simulink model "ANCwithError"  (R2023b)
settings: Solver=VariableStepAuto  StartTime=0.0  StopTime=10.0  RelTol=1e-3
libraries: matrix_library x54, dspadpt3 x30, raspberrypiAVlib x2, dspfdesign x2, audiosources x1
(part 2 of 2)

== system ANCwithError/Audio Processing/Subsystem2/Subsystem4 ==
  In1 : Inport
  In2 : Inport  Port=2
  Constant : Constant  Value=0.5
  Delay1 : Delay  DelayLength=1
  Estim. sec. path : DiscreteFir  Commented=through  Coefficients="[0.466  0.533  -0.257  -0.274  -0.231  -0.175]"
  Gain : Gain  Gain=-1
  LMS Update : dspadpt3/LMS Update  Method=Normalized LMS  Length=200  NumFilters=1  StepSizeSource=Input port  StepSize=0.1  LeakageFactor=1.0  InitialConditions=0  AdaptiveFilterMode=Tapped delay-line FIR filter  EnableAdaptInput=off  EnableResetInput=off  SimulateUsing=Interpreted execution
  LMS filter copy : DiscreteFir  CoefSource=Input port
      settings: InputPortMap=u0,u1
  y : Outport
  wires:
  Gain/1 -> y/1
  Constant/1 -> LMS Update/3
  LMS filter copy/1 -> Gain/1
  [coefs] -> LMS filter copy/2
  Delay1/1 -> [coefs]
  LMS Update/1 -> Delay1/1
  In1/1 -> Estim. sec. path/1, LMS filter copy/1
  Estim. sec. path/1 -> LMS Update/1
  In2/1 -> LMS Update/2

== system ANCwithError/Audio Processing/Subsystem2/Subsystem5 ==
  In1 : Inport
  In2 : Inport  Port=2
  Constant : Constant  Value=0.5
  Delay1 : Delay  DelayLength=1
  Estim. sec. path : DiscreteFir  Commented=through  Coefficients="[0.466  0.533  -0.257  -0.274  -0.231  -0.175]"
  Gain : Gain  Gain=-1
  LMS Update : dspadpt3/LMS Update  Method=Normalized LMS  Length=200  NumFilters=1  StepSizeSource=Input port  StepSize=0.1  LeakageFactor=1.0  InitialConditions=0  AdaptiveFilterMode=Tapped delay-line FIR filter  EnableAdaptInput=off  EnableResetInput=off  SimulateUsing=Interpreted execution
  LMS filter copy : DiscreteFir  CoefSource=Input port
      settings: InputPortMap=u0,u1
  y : Outport
  wires:
  Gain/1 -> y/1
  Constant/1 -> LMS Update/3
  LMS filter copy/1 -> Gain/1
  [coefs] -> LMS filter copy/2
  Delay1/1 -> [coefs]
  LMS Update/1 -> Delay1/1
  In1/1 -> Estim. sec. path/1, LMS filter copy/1
  Estim. sec. path/1 -> LMS Update/1
  In2/1 -> LMS Update/2

== system ANCwithError/Audio Processing/Subsystem2/Subsystem6 ==
  In1 : Inport
  In2 : Inport  Port=2
  Constant : Constant  Value=0.5
  Delay1 : Delay  DelayLength=1
  Estim. sec. path : DiscreteFir  Commented=through  Coefficients="[0.466  0.533  -0.257  -0.274  -0.231  -0.175]"
  Gain : Gain  Gain=-1
  LMS Update : dspadpt3/LMS Update  Method=Normalized LMS  Length=200  NumFilters=1  StepSizeSource=Input port  StepSize=0.1  LeakageFactor=1.0  InitialConditions=0  AdaptiveFilterMode=Tapped delay-line FIR filter  EnableAdaptInput=off  EnableResetInput=off  SimulateUsing=Interpreted execution
  LMS filter copy : DiscreteFir  CoefSource=Input port
      settings: InputPortMap=u0,u1
  y : Outport
  wires:
  Gain/1 -> y/1
  Constant/1 -> LMS Update/3
  LMS filter copy/1 -> Gain/1
  [coefs] -> LMS filter copy/2
  Delay1/1 -> [coefs]
  LMS Update/1 -> Delay1/1
  In1/1 -> Estim. sec. path/1, LMS filter copy/1
  Estim. sec. path/1 -> LMS Update/1
  In2/1 -> LMS Update/2

== system ANCwithError/Audio Processing/Subsystem2/Subsystem7 ==
  note: Anti-noise
  In1 : Inport
  In2 : Inport  Port=2
  Constant : Constant  Value=0.5
  Delay1 : Delay  DelayLength=1
  Estim. sec. path : DiscreteFir  Commented=through  Coefficients="[0.466  0.533  -0.257  -0.274  -0.231  -0.175]"
  Gain : Gain  Gain=-1
  LMS Update : dspadpt3/LMS Update  Method=Normalized LMS  Length=200  NumFilters=1  StepSizeSource=Input port  StepSize=0.1  LeakageFactor=1.0  InitialConditions=0  AdaptiveFilterMode=Tapped delay-line FIR filter  EnableAdaptInput=off  EnableResetInput=off  SimulateUsing=Interpreted execution
  LMS filter copy : DiscreteFir  CoefSource=Input port
      settings: InputPortMap=u0,u1
  y : Outport
  wires:
  Gain/1 -> y/1
  Constant/1 -> LMS Update/3
  LMS filter copy/1 -> Gain/1
  [coefs] -> LMS filter copy/2
  Delay1/1 -> [coefs]
  LMS Update/1 -> Delay1/1
  In1/1 -> Estim. sec. path/1, LMS filter copy/1
  Estim. sec. path/1 -> LMS Update/1
  In2/1 -> LMS Update/2

== system ANCwithError/Audio Processing/Subsystem2/Subsystem8 ==
  note: Anti-noise
  In1 : Inport
  In2 : Inport  Port=2
  Constant : Constant  Value=0.5
  Delay1 : Delay  DelayLength=1
  Estim. sec. path : DiscreteFir  Commented=through  Coefficients="[0.466  0.533  -0.257  -0.274  -0.231  -0.175]"
  Gain : Gain  Gain=-1
  LMS Update : dspadpt3/LMS Update  Method=Normalized LMS  Length=200  NumFilters=1  StepSizeSource=Input port  StepSize=0.1  LeakageFactor=1.0  InitialConditions=0  AdaptiveFilterMode=Tapped delay-line FIR filter  EnableAdaptInput=off  EnableResetInput=off  SimulateUsing=Interpreted execution
  LMS filter copy : DiscreteFir  CoefSource=Input port
      settings: InputPortMap=u0,u1
  y : Outport
  wires:
  Gain/1 -> y/1
  Constant/1 -> LMS Update/3
  LMS filter copy/1 -> Gain/1
  [coefs] -> LMS filter copy/2
  Delay1/1 -> [coefs]
  LMS Update/1 -> Delay1/1
  In1/1 -> Estim. sec. path/1, LMS filter copy/1
  Estim. sec. path/1 -> LMS Update/1
  In2/1 -> LMS Update/2

== system ANCwithError/Audio Processing/Subsystem2/Subsystem9 ==
  note: Anti-noise
  In1 : Inport
  In2 : Inport  Port=2
  Constant : Constant  Value=0.5
  Delay1 : Delay  DelayLength=1
  Estim. sec. path : DiscreteFir  Commented=through  Coefficients="[0.466  0.533  -0.257  -0.274  -0.231  -0.175]"
  Gain : Gain  Gain=-1
  LMS Update : dspadpt3/LMS Update  Method=Normalized LMS  Length=200  NumFilters=1  StepSizeSource=Input port  StepSize=0.1  LeakageFactor=1.0  InitialConditions=0  AdaptiveFilterMode=Tapped delay-line FIR filter  EnableAdaptInput=off  EnableResetInput=off  SimulateUsing=Interpreted execution
  LMS filter copy : DiscreteFir  CoefSource=Input port
      settings: InputPortMap=u0,u1
  y : Outport
  wires:
  Gain/1 -> y/1
  Constant/1 -> LMS Update/3
  LMS filter copy/1 -> Gain/1
  [coefs] -> LMS filter copy/2
  Delay1/1 -> [coefs]
  LMS Update/1 -> Delay1/1
  In1/1 -> Estim. sec. path/1, LMS filter copy/1
  Estim. sec. path/1 -> LMS Update/1
  In2/1 -> LMS Update/2
